simulink model "Maglev_14AE30004"  (Simulink 8.5)
settings: Solver=ode45  StartTime=0.0  StopTime=10.0  RelTol=1e-3
libraries: simulink x4
settings Model: Creator=Aranya Dan  LastModifiedBy=Aranya Dan
settings DataIOCC: SignalLoggingSaveFormat=Dataset
settings OptimizationCC: ExpressionDepthLimit=128
settings DebuggingCC: UnderspecifiedInitializationDetection=Simplified  MergeDetectMultiDrivingBlocksExec=error  FcnCallInpInsideContextMsg=EnableAllAsError  StateNameClashWarn=none
settings GRTTargetCC: CombineOutputUpdateFcns=on  GRTInterface=off

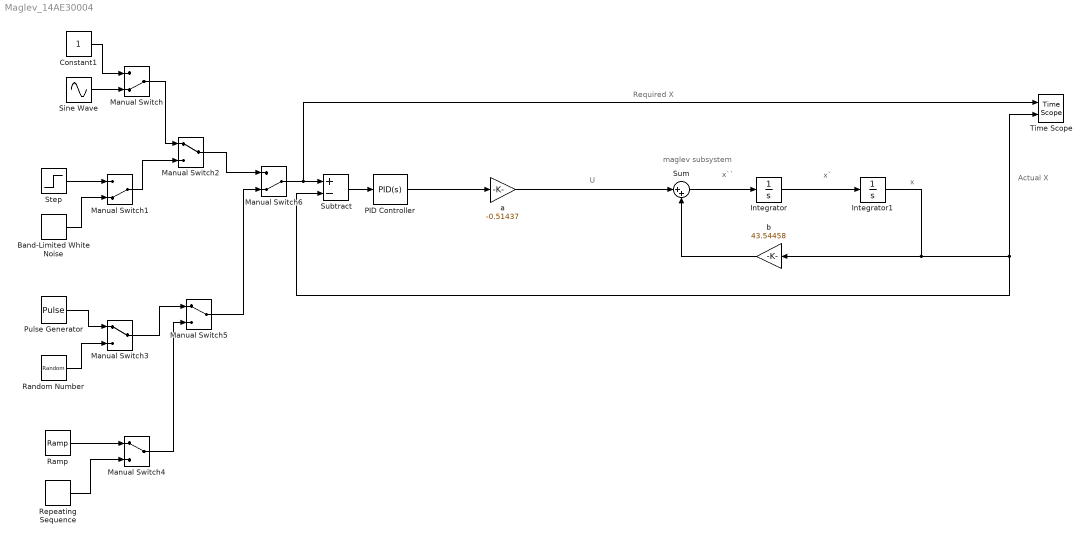
== system Maglev_14AE30004 ==
  note: Actual X
  note: Required X
  note: maglev subsystem
  note: U
  note: x`
  note: x``
  note: x
  Band-Limited White Noise : simulink/Sources/Band-Limited White Noise  Cov=[0.1]  Ts=0.1  seed=[23341]
  Constant1 : Constant
  Integrator : Integrator
  Integrator1 : Integrator
  Manual Switch : ManualSwitch  CurrentSetting=0
  Manual Switch1 : ManualSwitch  CurrentSetting=0
  Manual Switch{2..5} (4 alike) : ManualSwitch
  Manual Switch6 : ManualSwitch  CurrentSetting=0
  PID Controller : simulink/Continuous/PID Controller  Controller=PID  TimeDomain=Continuous-time  SampleTime=-1  IntegratorMethod=Forward Euler  FilterMethod=Forward Euler  Form=Parallel  UseFilter=on  ControllerParametersSource=internal  P=-1802.72408045143  I=-5937.87773793035  D=-134.391115123266  N=383.735329400122  InitialConditionSource=internal  InitialConditionForIntegrator=0  InitialConditionForFilter=0  ExternalReset=none  LimitOutput=off  UpperSaturationLimit=inf  LowerSaturationLimit=-inf  LinearizeAsGain=on  AntiWindupMode=none  Kb=1  TrackingMode=off  Kt=1  PParamMin=[]  PParamMax=[]  IParamMin=[]  IParamMax=[]  DParamMin=[]  DParamMax=[]  NParamMin=[]  NParamMax=[]  KbParamMin=[]  KbParamMax=[]  KtParamMin=[]  KtParamMax=[]  POutMin=[]  POutMax=[]  IOutMin=[]  IOutMax=[]  DOutMin=[]  DOutMax=[]  NOutMin=[]  NOutMax=[]  KbOutMin=[]  KbOutMax=[]  KtOutMin=[]  KtOutMax=[]  IntegratorOutMin=[]  IntegratorOutMax=[]  FilterOutMin=[]  FilterOutMax=[]  SumOutMin=[]  SumOutMax=[]  SumI1OutMin=[]  SumI1OutMax=[]  SumI2OutMin=[]  SumI2OutMax=[]  SumI3OutMin=[]  SumI3OutMax=[]  SumDOutMin=[]  SumDOutMax=[]  SaturationOutMin=[]  SaturationOutMax=[]  IntegratorContinuousStateAttributes=''  IntegratorStateMustResolveToSignalObject=off  IntegratorRTWStateStorageClass=Auto  FilterContinuousStateAttributes=''  FilterStateMustResolveToSignalObject=off  FilterRTWStateStorageClass=Auto  DifferentiatorICPrevScaledInput=0  DifferentiatorOutMin=[]  DifferentiatorOutMax=[]
  Pulse Generator : DiscretePulseGenerator  PulseType=Time based  Period=10  PulseWidth=5
  Ramp : simulink/Sources/Ramp  slope=1  start=0  X0=0
  Random Number : RandomNumber  SampleTime=0.1
  Repeating Sequence : simulink/Sources/Repeating Sequence  rep_seq_t=[0 2]  rep_seq_y=[0 2]
  Sine Wave : Sin  SampleTime=0
  Step : Step  SampleTime=0
  Subtract : Sum  Inputs=+-
  Sum : Sum  Inputs=|++
  Time Scope : TimeScope  DefaultConfigurationName=spbscopes.TimeScopeBlockCfg  NumInputPorts=2
  a : Gain  Gain=-0.51437
  b : Gain  Gain=43.54458
  wires:
  Band-Limited White Noise/1 -> Manual Switch1/2
  Manual Switch1/1 -> Manual Switch2/2
  Constant1/1 -> Manual Switch/1
  Step/1 -> Manual Switch1/1
  Manual Switch/1 -> Manual Switch2/1
  Sine Wave/1 -> Manual Switch/2
  PID Controller/1 -> a/1
  Subtract/1 -> PID Controller/1
  Integrator1/1 -> Subtract/2, Time Scope/2, b/1
  a/1 -> Sum/1
  Sum/1 -> Integrator/1
  Integrator/1 -> Integrator1/1
  b/1 -> Sum/2
  Pulse Generator/1 -> Manual Switch3/1
  Random Number/1 -> Manual Switch3/2
  Ramp/1 -> Manual Switch4/1
  Repeating Sequence/1 -> Manual Switch4/2
  Manual Switch4/1 -> Manual Switch5/2
  Manual Switch3/1 -> Manual Switch5/1
  Manual Switch6/1 -> Time Scope/1, Subtract/1
  Manual Switch5/1 -> Manual Switch6/2
  Manual Switch2/1 -> Manual Switch6/1
